simulink model "ConeInteractor"  (Simulink 6.6)
settings: Solver=FixedStepDiscrete  StartTime=0.0  StopTime=inf  FixedStep=0.1  RelTol=1e-3
libraries: SimvtkRenderingLibrary x5, SimvtkGraphicsLibrary x1
settings Model: Creator=dgobbi  LastModifiedBy=dgobbi

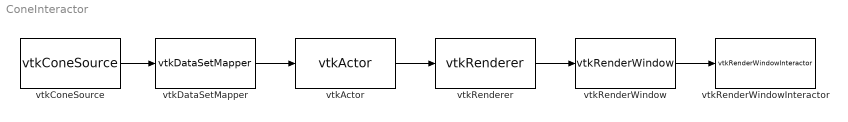
== system ConeInteractor ==
  vtkActor : SimvtkRenderingLibrary/vtkActor  VTKInputSelf=off  VTKInputBackfaceProperty=off  VTKInputMapper=on  VTKInputProperty=off  VTKInputTexture=off  VTKInputUserMatrix=off  VTKInputUserTransform=off  DragableInputIndicator=Use Default  VTKParamDragable=0  OrientationInputIndicator=Use Default  VTKParamOrientation=[0,0,0]  OriginInputIndicator=Use Default  VTKParamOrigin=[0,0,0]  PickableInputIndicator=Use Default  VTKParamPickable=0  PositionInputIndicator=Use Default  VTKParamPosition=[0,0,0]  ScaleInputIndicator=Use Default  VTKParamScale=[0,0,0]  VisibilityInputIndicator=Use Default  VTKParamVisibility=0  VTKOutputSelf=on  VTKOutputMatrix=off  VTKOutputNextPart=off  VTKOutputNextPath=off
  vtkConeSource : SimvtkGraphicsLibrary/vtkConeSource  AngleInputIndicator=Use Default  VTKParamAngle=0  CappingInputIndicator=Use Default  VTKParamCapping=0  CenterInputIndicator=Use Default  VTKParamCenter=[0,0,0]  DirectionInputIndicator=Use Default  VTKParamDirection=[0,0,0]  HeightInputIndicator=Use Default  VTKParamHeight=0  RadiusInputIndicator=Use Default  VTKParamRadius=0  ResolutionInputIndicator=Use Default  VTKParamResolution=0  VTKOutputSelf=off
  vtkDataSetMapper : SimvtkRenderingLibrary/vtkDataSetMapper  VTKInputSelf=off  VTKInputClippingPlane=0  VTKInputClippingPlanes=off  VTKInputLookupTable=off  ColorModeInputIndicator=Use Default  VTKParamColorMode=0  ImmediateModeRenderingInputIndicator=Use Default  VTKParamImmediateModeRendering=0  InterpolateScalarsBeforeMappingInputIndicator=Use Default  VTKParamInterpolateScalarsBeforeMapping=0  RenderTimeInputIndicator=Use Default  VTKParamRenderTime=0  ScalarMaterialModeInputIndicator=Use Default  VTKParamScalarMaterialMode=0  ScalarModeInputIndicator=Use Default  VTKParamScalarMode=0  ScalarRangeInputIndicator=Use Default  VTKParamScalarRange=[0,0]  ScalarVisibilityInputIndicator=Use Default  VTKParamScalarVisibility=0  StaticInputIndicator=Use Default  VTKParamStatic=0  UseLookupTableScalarRangeInputIndicator=Use Default  VTKParamUseLookupTableScalarRange=0  VTKOutputSelf=on  VTKOutputPolyDataMapper=off
  vtkRenderWindow : SimvtkRenderingLibrary/vtkRenderWindow  VTKInputSelf=off  VTKInputInteractor=off  VTKInputRenderer=1  AAFramesInputIndicator=Use Default  VTKParamAAFrames=0  AbortRenderInputIndicator=Use Default  VTKParamAbortRender=0  AlphaBitPlanesInputIndicator=Use Default  VTKParamAlphaBitPlanes=0  AnaglyphColorMaskInputIndicator=Use Default  VTKParamAnaglyphColorMask=[0,0]  AnaglyphColorSaturationInputIndicator=Use Default  VTKParamAnaglyphColorSaturation=0  BordersInputIndicator=Use Default  VTKParamBorders=0  CurrentCursorInputIndicator=Use Default  VTKParamCurrentCursor=0  DPIInputIndicator=Use Default  VTKParamDPI=0  DesiredUpdateRateInputIndicator=Use Default  VTKParamDesiredUpdateRate=0  DoubleBufferInputIndicator=Use Default  VTKParamDoubleBuffer=0  EraseInputIndicator=Use Default  VTKParamErase=0  FDFramesInputIndicator=Use Default  VTKParamFDFrames=0  FullScreenInputIndicator=Use Default  VTKParamFullScreen=0  InAbortCheckInputIndicator=Use Default  VTKParamInAbortCheck=0  IsPickingInputIndicator=Use Default  VTKParamIsPicking=0  LineSmoothingInputIndicator=Use Default  VTKParamLineSmoothing=0  MappedInputIndicator=Use Default  VTKParamMapped=0  MultiSamplesInputIndicator=Use Default  VTKParamMultiSamples=0  NumberOfLayersInputIndicator=Use Default  VTKParamNumberOfLayers=0  OffScreenRenderingInputIndicator=Use Default  VTKParamOffScreenRendering=0  PointSmoothingInputIndicator=Use Default  VTKParamPointSmoothing=0  PolygonSmoothingInputIndicator=Use Default  VTKParamPolygonSmoothing=0  PositionInputIndicator=Use Default  VTKParamPosition=[0,0]  ReportGraphicErrorsInputIndicator=Use Default  VTKParamReportGraphicErrors=0  SizeInputIndicator=Use Default  VTKParamSize=[0,0]  StencilCapableInputIndicator=Use Default  VTKParamStencilCapable=0  StereoCapableWindowInputIndicator=Use Default  VTKParamStereoCapableWindow=0  StereoRenderInputIndicator=Use Default  VTKParamStereoRender=0  StereoTypeInputIndicator=Use Default  VTKParamStereoType=0  SubFramesInputIndicator=Use Default  VTKParamSubFrames=0  SwapBuffersInputIndicator=Use Default  VTKParamSwapBuffers=0  TileScaleInputIndicator=Use Default  VTKParamTileScale=[0,0]  TileViewportInputIndicator=Use Default  VTKParamTileViewport=[0,0,0,0]  WindowNameInputIndicator=Use Default  VTKParamWindowName=0  VTKOutputSelf=on  VTKOutputPainterDeviceAdapter=off  VTKOutputRenderers=off
  vtkRenderWindowInteractor : SimvtkRenderingLibrary/vtkRenderWindowInteractor  VTKInputSelf=off  VTKInputInteractorStyle=off  VTKInputPicker=off  VTKInputRenderWindow=on  AltKeyInputIndicator=Use Default  VTKParamAltKey=0  ControlKeyInputIndicator=Use Default  VTKParamControlKey=0  DesiredUpdateRateInputIndicator=Use Default  VTKParamDesiredUpdateRate=0  DollyInputIndicator=Use Default  VTKParamDolly=0  EventPositionInputIndicator=Use Default  VTKParamEventPosition=[0,0]  EventSizeInputIndicator=Use Default  VTKParamEventSize=[0,0]  KeyCodeInputIndicator=Use Default  VTKParamKeyCode=0  KeySymInputIndicator=Use Default  VTKParamKeySym=0  LastEventPositionInputIndicator=Use Default  VTKParamLastEventPosition=[0,0]  LightFollowCameraInputIndicator=Use Default  VTKParamLightFollowCamera=0  NumberOfFlyFramesInputIndicator=Use Default  VTKParamNumberOfFlyFrames=0  RepeatCountInputIndicator=Use Default  VTKParamRepeatCount=0  ShiftKeyInputIndicator=Use Default  VTKParamShiftKey=0  SizeInputIndicator=Use Default  VTKParamSize=[0,0]  StillUpdateRateInputIndicator=Use Default  VTKParamStillUpdateRate=0  TimerDurationInputIndicator=Use Default  VTKParamTimerDuration=0  TimerEventDurationInputIndicator=Use Default  VTKParamTimerEventDuration=0  TimerEventIdInputIndicator=Use Default  VTKParamTimerEventId=0  TimerEventPlatformIdInputIndicator=Use Default  VTKParamTimerEventPlatformId=0  TimerEventTypeInputIndicator=Use Default  VTKParamTimerEventType=0  VTKOutputSelf=off  VTKOutputObserverMediator=off
  vtkRenderer : SimvtkRenderingLibrary/vtkRenderer  VTKInputSelf=off  VTKInputActiveCamera=off  VTKInputActor=1  VTKInputActor2D=0  VTKInputCuller=0  VTKInputLight=0  VTKInputProp=0  VTKInputViewProp=0  VTKInputVolume=0  AllocatedRenderTimeInputIndicator=Use Default  VTKParamAllocatedRenderTime=0  AmbientInputIndicator=Use Default  VTKParamAmbient=[0,0,0]  AspectInputIndicator=Use Default  VTKParamAspect=[0,0]  AutomaticLightCreationInputIndicator=Use Default  VTKParamAutomaticLightCreation=0  BackgroundInputIndicator=Use Default  VTKParamBackground=[0,0,0]  Background2InputIndicator=Use Default  VTKParamBackground2=[0,0,0]  BackingStoreInputIndicator=Use Default  VTKParamBackingStore=0  DisplayPointInputIndicator=Use Default  VTKParamDisplayPoint=[0,0,0]  DrawInputIndicator=Use Default  VTKParamDraw=0  EraseInputIndicator=Use Default  VTKParamErase=0  GradientBackgroundInputIndicator=Use Default  VTKParamGradientBackground=0  InteractiveInputIndicator=Use Default  VTKParamInteractive=0  LayerInputIndicator=Use Default  VTKParamLayer=0  LightFollowCameraInputIndicator=Use Default  VTKParamLightFollowCamera=0  MaximumNumberOfPeelsInputIndicator=Use Default  VTKParamMaximumNumberOfPeels=0  NearClippingPlaneToleranceInputIndicator=Use Default  VTKParamNearClippingPlaneTolerance=0  OcclusionRatioInputIndicator=Use Default  VTKParamOcclusionRatio=0  PixelAspectInputIndicator=Use Default  VTKParamPixelAspect=[0,0]  TwoSidedLightingInputIndicator=Use Default  VTKParamTwoSidedLighting=0  UseDepthPeelingInputIndicator=Use Default  VTKParamUseDepthPeeling=0  ViewPointInputIndicator=Use Default  VTKParamViewPoint=[0,0,0]  ViewportInputIndicator=Use Default  VTKParamViewport=[0,0,0,0]  WorldPointInputIndicator=Use Default  VTKParamWorldPoint=[0,0,0,0]  VTKOutputSelf=on  VTKOutputActors=off  VTKOutputActors2D=off  VTKOutputCullers=off  VTKOutputLights=off  VTKOutputPickResultProps=off  VTKOutputProps=off  VTKOutputVTKWindow=off  VTKOutputViewProps=off  VTKOutputVolumes=off
  wires:
  vtkConeSource/1 -> vtkDataSetMapper/1
  vtkDataSetMapper/1 -> vtkActor/1
  vtkActor/1 -> vtkRenderer/1
  vtkRenderer/1 -> vtkRenderWindow/1
  vtkRenderWindow/1 -> vtkRenderWindowInteractor/1
